simulink model "Parametri_PIDa"  (R2015b)
settings: Solver=VariableStepAuto  StartTime=0.0  StopTime=50  RelTol=1e-3
libraries: simulink x1
settings Model: Creator=User  LastModifiedBy=User

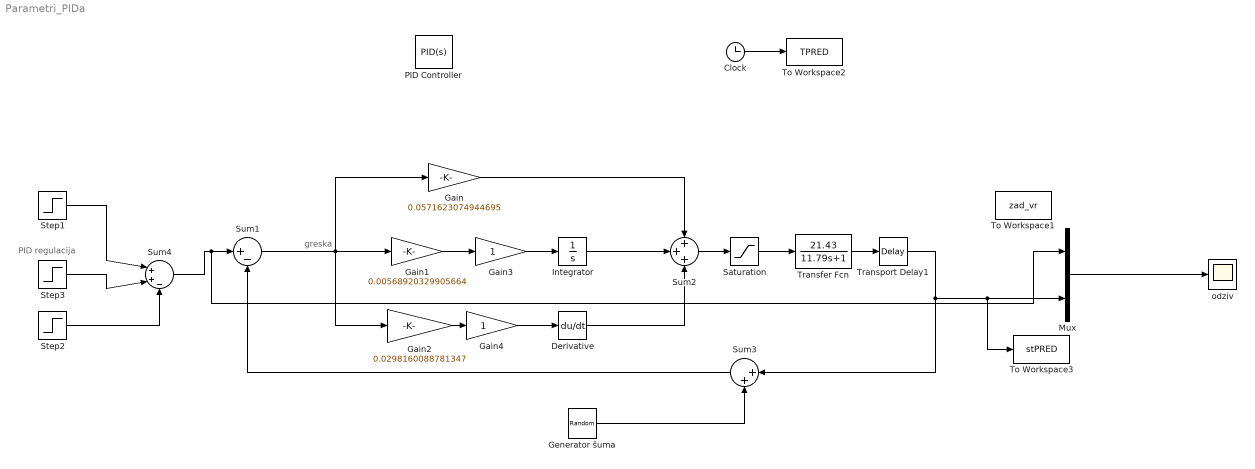
== system Parametri_PIDa ==
  note: greska
  note: PID regulacija
  Clock : Clock
  Derivative : Derivative
  Gain : Gain  Gain=0.0571623074944695
  Gain1 : Gain  Gain=0.00568920329905664
  Gain2 : Gain  Gain=0.0298160088781347
  Gain3 : Gain
  Gain4 : Gain
  Generator šuma : UniformRandomNumber  Minimum=0  Maximum=0.18  Seed=1  SampleTime=0.01
  Integrator : Integrator  LimitOutput=on  UpperSaturationLimit=10  LowerSaturationLimit=0
  Mux : Mux  Inputs=2
  PID Controller : simulink/Continuous/PID Controller  Controller=PID  TimeDomain=Continuous-time  SampleTime=-1  IntegratorMethod=Forward Euler  FilterMethod=Forward Euler  Form=Parallel  UseFilter=on  ControllerParametersSource=internal  P=0.0571623074944695  I=0.00568920329905664  D=0.0298160088781347  N=0.296180832075482  InitialConditionSource=internal  InitialConditionForIntegrator=0  InitialConditionForFilter=0  ExternalReset=level  LimitOutput=off  UpperSaturationLimit=inf  LowerSaturationLimit=-inf  LinearizeAsGain=on  AntiWindupMode=none  Kb=1  TrackingMode=off  Kt=1  PParamMin=[]  PParamMax=[]  IParamMin=[]  IParamMax=[]  DParamMin=[]  DParamMax=[]  NParamMin=[]  NParamMax=[]  KbParamMin=[]  KbParamMax=[]  KtParamMin=[]  KtParamMax=[]  POutMin=[]  POutMax=[]  IOutMin=[]  IOutMax=[]  DOutMin=[]  DOutMax=[]  NOutMin=[]  NOutMax=[]  KbOutMin=[]  KbOutMax=[]  KtOutMin=[]  KtOutMax=[]  IntegratorOutMin=[]  IntegratorOutMax=[]  FilterOutMin=[]  FilterOutMax=[]  SumOutMin=[]  SumOutMax=[]  SumI1OutMin=[]  SumI1OutMax=[]  SumI2OutMin=[]  SumI2OutMax=[]  SumI3OutMin=[]  SumI3OutMax=[]  SumDOutMin=[]  SumDOutMax=[]  SaturationOutMin=[]  SaturationOutMax=[]  IntegratorContinuousStateAttributes=''  IntegratorStateMustResolveToSignalObject=off  IntegratorRTWStateStorageClass=Auto  FilterContinuousStateAttributes=''  FilterStateMustResolveToSignalObject=off  FilterRTWStateStorageClass=Auto  DifferentiatorICPrevScaledInput=0  DifferentiatorOutMin=[]  DifferentiatorOutMax=[]
  Saturation : Saturate  UpperLimit=10  LowerLimit=0
  Step1 : Step  After=60  SampleTime=0
  Step2 : Step  Time=25  After=20  SampleTime=0
  Step3 : Step  Time=15  After=50  SampleTime=0
  Sum1 : Sum  Inputs=|+-
  Sum2 : Sum  Inputs=+++
  Sum3 : Sum  Inputs=|++
  Sum4 : Sum  Inputs=|++-
  To Workspace1 : ToWorkspace  VariableName=zad_vr  SampleTime=-1
      settings: Save2DSignal=2-D array (concatenate along first dimension)
  To Workspace2 : ToWorkspace  VariableName=TPRED  SampleTime=-1
  To Workspace3 : ToWorkspace  VariableName=stPRED  SampleTime=-1
  Transfer Fcn : TransferFcn  Numerator=[21.43]  Denominator=[11.79 1]
  Transport Delay1 : TransportDelay  DelayTime=0.1
  "odziv " : Scope
  wires:
  Transfer Fcn/1 -> Transport Delay1/1
  Transport Delay1/1 -> Sum3/1, To Workspace3/1, Mux/2
  Gain/1 -> Sum2/1
  Clock/1 -> To Workspace2/1
  Saturation/1 -> Transfer Fcn/1
  Sum3/1 -> Sum1/2
  Generator šuma/1 -> Sum3/2
  Gain1/1 -> Gain3/1
  Gain2/1 -> Gain4/1
  Integrator/1 -> Sum2/2
  Derivative/1 -> Sum2/3
  Mux/1 -> "odziv "/1
  Gain3/1 -> Integrator/1
  Gain4/1 -> Derivative/1
  Step3/1 -> Sum4/2
  Step2/1 -> Sum4/3
  Step1/1 -> Sum4/1
  Sum4/1 -> Mux/1, Sum1/1
  Sum1/1 -> Gain2/1, Gain/1, Gain1/1
  Sum2/1 -> Saturation/1
